simulink library "provalibrary"  (R2023b)
settings: Solver=VariableStepAuto  StartTime=0.0  StopTime=10.0  RelTol=1e-3
values from neighbouring files (symbols this model uses):
  A0 = [0 1 0; 0 0 1; 1, 0, 0]    [data_38.m]
  P = F_e / c    [data_38.m]
libraries: matrix_library x2, sharedutil x1
settings Model: Creator=alexb  LastModifiedBy=alexb
settings OptimizationCC: ReuseModelBlockBuffer=off

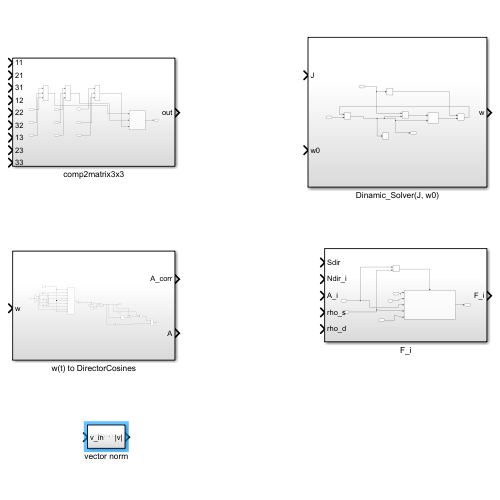
[thumbnail: Simulink's stored preview of the top-level diagram]
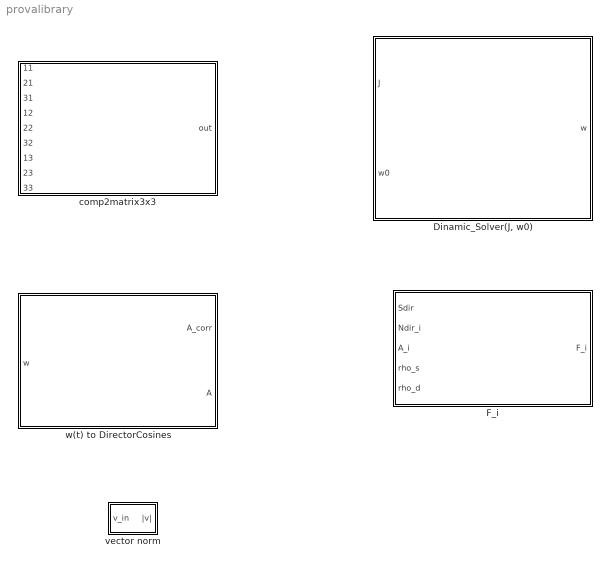
== system provalibrary ==
  "Dinamic_Solver(J, w0)" : Subsystem
  F_i : Subsystem
  comp2matrix3x3 : Subsystem
  vector norm : Subsystem
  w(t) to DirectorCosines : Subsystem

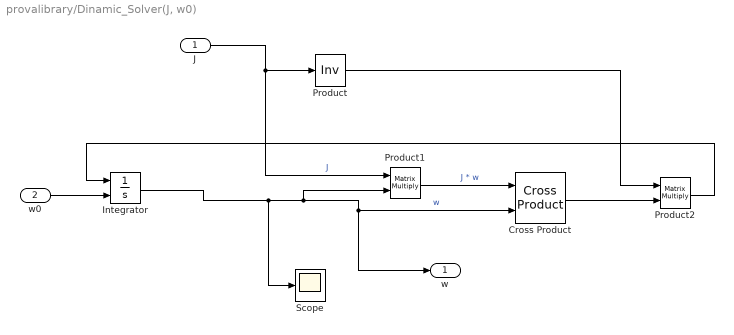
== system provalibrary/Dinamic_Solver(J, w0) ==
  J : Inport
  w0 : Inport  Port=2
  Cross Product : matrix_library/Cross Product
  Integrator : Integrator  InitialConditionSource=external
  Product : Product  Inputs=/  Multiplication=Matrix(*)
  Product1 : Product  Multiplication=Matrix(*)
  Product2 : Product  Multiplication=Matrix(*)
  Scope : Scope
  w : Outport
  wires:
  Product/1 -> Product2/1
  Product2/1 -> Integrator/1
  J/1 -> Product1/1, Product/1  "J"
  Integrator/1 -> w/1, Cross Product/2, Product1/2, Scope/1  "w"
  Product1/1 -> Cross Product/1  "J * w"
  w0/1 -> Integrator/2
  Cross Product/1 -> Product2/2

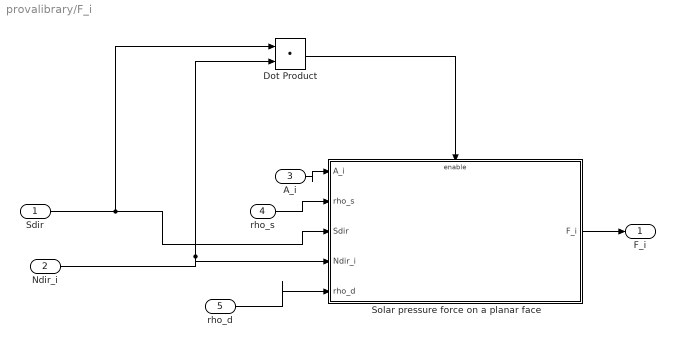
== system provalibrary/F_i ==
  Sdir : Inport
  Ndir_i : Inport  Port=2
  A_i : Inport  Port=3
  rho_s : Inport  Port=4
  rho_d : Inport  Port=5
  Dot Product : DotProduct  OutDataTypeStr=Inherit: Inherit via internal rule
  Solar pressure force on a planar face : Subsystem  TreatAsAtomicUnit=on
  F_i : Outport
  wires:
  Dot Product/1 -> Solar pressure force on a planar face/Enable
  Sdir/1 -> Dot Product/1, Solar pressure force on a planar face/3(Sdir)
  Ndir_i/1 -> Dot Product/2, Solar pressure force on a planar face/4(Ndir_i)
  rho_s/1 -> Solar pressure force on a planar face/2(rho_s)
  A_i/1 -> Solar pressure force on a planar face/1(A_i)
  rho_d/1 -> Solar pressure force on a planar face/5(rho_d)
  Solar pressure force on a planar face/1(F_i) -> F_i/1

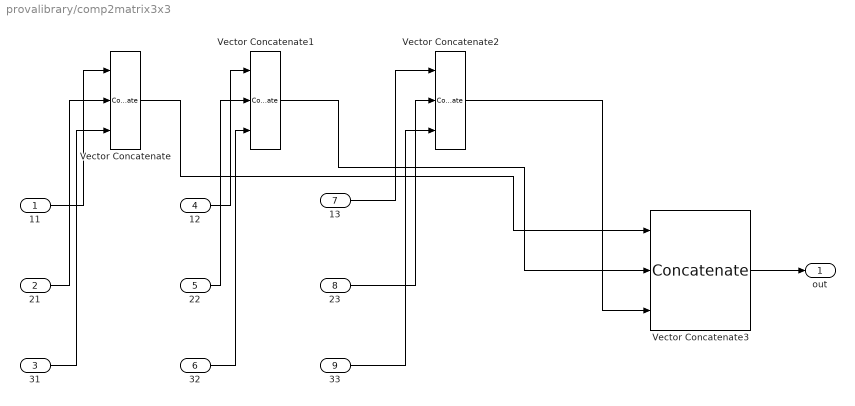
== system provalibrary/comp2matrix3x3 ==
  11 : Inport
  21 : Inport  Port=2
  31 : Inport  Port=3
  12 : Inport  Port=4
  22 : Inport  Port=5
  32 : Inport  Port=6
  13 : Inport  Port=7
  23 : Inport  Port=8
  33 : Inport  Port=9
  Vector Concatenate : Concatenate  NumInputs=3
  Vector Concatenate1 : Concatenate  NumInputs=3
  Vector Concatenate2 : Concatenate  NumInputs=3
  Vector Concatenate3 : Concatenate  NumInputs=3  Mode=Multidimensional array  ConcatenateDimension=2
  out : Outport
  wires:
  11/1 -> Vector Concatenate/1
  Vector Concatenate1/1 -> Vector Concatenate3/2
  Vector Concatenate/1 -> Vector Concatenate3/1
  31/1 -> Vector Concatenate/3
  13/1 -> Vector Concatenate2/1
  23/1 -> Vector Concatenate2/2
  Vector Concatenate2/1 -> Vector Concatenate3/3
  21/1 -> Vector Concatenate/2
  12/1 -> Vector Concatenate1/1
  22/1 -> Vector Concatenate1/2
  32/1 -> Vector Concatenate1/3
  33/1 -> Vector Concatenate2/3
  Vector Concatenate3/1 -> out/1

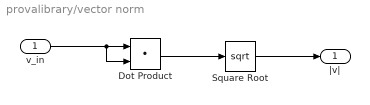
== system provalibrary/vector norm ==
  v_in : Inport
  Dot Product : DotProduct  OutDataTypeStr=Inherit: Inherit via internal rule
  Square Root : Sqrt
  |v| : Outport
  wires:
  v_in/1 -> Dot Product/2, Dot Product/1
  Dot Product/1 -> Square Root/1
  Square Root/1 -> |v|/1

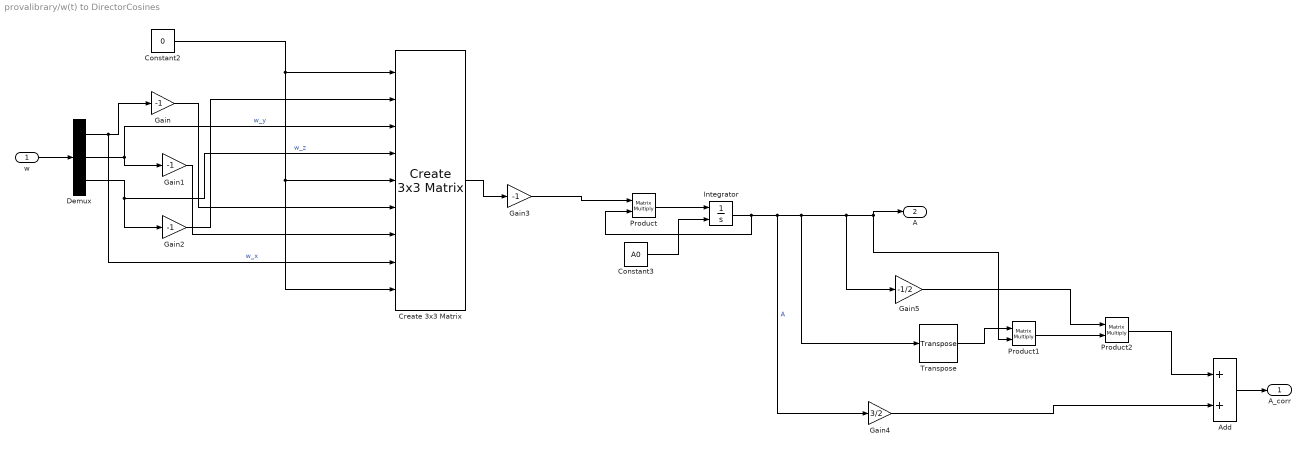
== system provalibrary/w(t) to DirectorCosines ==
  w : Inport
  Add : Sum
  Constant2 : Constant  Value=0
  Constant3 : Constant  Value=A0
  Create 3x3 Matrix : sharedutil/Create 3x3 Matrix  aMode=aMode
      settings: LibrarySourceBlock=aerolibutil/Create 3x3 Matrix
  Demux : Demux  Outputs=3
  Gain{,1..3} (4 alike) : Gain  Gain=-1
  Gain4 : Gain  Gain=3/2
  Gain5 : Gain  Gain=-1/2
  Integrator : Integrator  InitialConditionSource=external
  Product : Product  Multiplication=Matrix(*)
  Product1 : Product  Multiplication=Matrix(*)
  Product2 : Product  Multiplication=Matrix(*)
  Transpose : matrix_library/Transpose
  A_corr : Outport
  A : Outport  Port=2
  wires:
  Gain1/1 -> Create 3x3 Matrix/7
  Gain5/1 -> Product2/1
  Product1/1 -> Product2/2
  Transpose/1 -> Product1/1
  Gain4/1 -> Add/2
  Product2/1 -> Add/1
  Constant3/1 -> Integrator/2
  Demux/1 -> Create 3x3 Matrix/8, Gain/1  "w_x"
  Gain/1 -> Create 3x3 Matrix/6
  Constant2/1 -> Create 3x3 Matrix/9, Create 3x3 Matrix/5, Create 3x3 Matrix/1
  Add/1 -> A_corr/1
  Product/1 -> Integrator/1
  Demux/3 -> Create 3x3 Matrix/4, Gain2/1  "w_z"
  Gain2/1 -> Create 3x3 Matrix/2
  Integrator/1 -> Product/2, Gain4/1, Transpose/1, Gain5/1, A/1, Product1/2  "A"
  Demux/2 -> Create 3x3 Matrix/3, Gain1/1  "w_y"
  w/1 -> Demux/1
  Create 3x3 Matrix/1 -> Gain3/1
  Gain3/1 -> Product/1

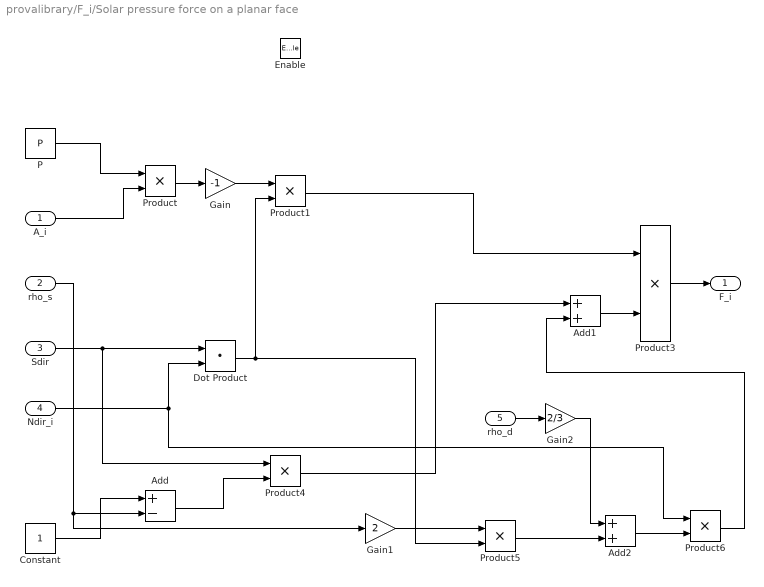
== system provalibrary/F_i/Solar pressure force on a planar face ==
  A_i : Inport
  rho_s : Inport  Port=2
  Sdir : Inport  Port=3
  Ndir_i : Inport  Port=4
  rho_d : Inport  Port=5
  Enable : EnablePort
  Add : Sum  Inputs=+-
  Add1 : Sum
  Add2 : Sum
  Constant : Constant
  Dot Product : DotProduct  OutDataTypeStr=Inherit: Inherit via internal rule
  Gain : Gain  Gain=-1
  Gain1 : Gain  Gain=2
  Gain2 : Gain  Gain=2/3
  P : Constant  Value=P
  Product{,1,3..6} (6 alike) : Product
  F_i : Outport
  wires:
  P/1 -> Product/1
  A_i/1 -> Product/2
  Product/1 -> Gain/1
  Gain/1 -> Product1/1
  Dot Product/1 -> Product5/2, Product1/2
  Sdir/1 -> Dot Product/1, Product4/1
  Ndir_i/1 -> Dot Product/2, Product6/1
  Product1/1 -> Product3/1
  Constant/1 -> Add/1
  rho_s/1 -> Gain1/1, Add/2
  Add/1 -> Product4/2
  Add1/1 -> Product3/2
  Product4/1 -> Add1/1
  Gain1/1 -> Product5/1
  Product5/1 -> Add2/2
  rho_d/1 -> Gain2/1
  Gain2/1 -> Add2/1
  Add2/1 -> Product6/2
  Product6/1 -> Add1/2
  Product3/1 -> F_i/1
